simulink model "speed_control_disc_mpc"  (R2024a)
settings: Solver=VariableStepAuto  StartTime=0.0  StopTime=150  MaxStep=0.01  RelTol=1e-3
values from neighbouring files (symbols this model uses):
  F_max = 15    [init.m]
  F_min = -15    [init.m]
  K = ki*tau - kd/tau    (= -49.7)    [init.m]
  k = 0.5    [init.m]
  kbc = 1/(kp+kd/tau)    (= 0.0142857142857)    [init.m]
  kd = 5    [init.m]
  ki = 3    [init.m]
  kp = 20    [init.m]
  m = 10    [init.m]
  T = 0.1    [init.m]
  tau = 0.1    [init.m]
undefined symbols (not defined in the file or in its folder): DiscIntNeverNeededParam
libraries: simulink x4, mpclib x1, SignalEditorBlockLib x1
settings Model: Creator=berto  LastModifiedBy=berto

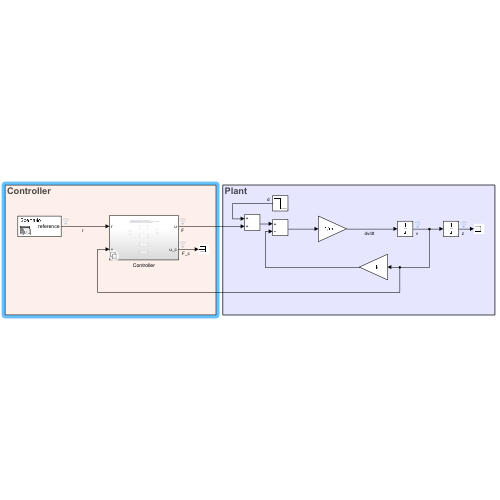
[thumbnail: Simulink's stored preview of the top-level diagram]
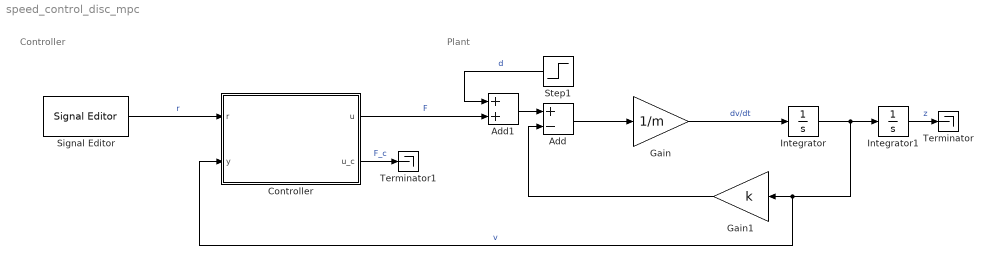
== system speed_control_disc_mpc ==
  note: Controller
  note: Plant
  Add : Sum  Inputs=+-
  Add1 : Sum
  Controller : Subsystem  Variant=on
  Gain : Gain  Gain=1/m
  Gain1 : Gain  Gain=k
  Integrator : Integrator
  Integrator1 : Integrator
  Signal Editor : SignalEditorBlockLib/Signal Editor  FileName=reference.mat  ActiveScenario=Scenario  ActiveSignal=reference  IsBus=off  OutputBusObjectStr=Bus: BusObject  SampleTime=0  ZeroCross=off  OutputAfterFinalValue=Setting to zero  Unit=inherit  PreserveSignalName=on  ApplySigPropsToAllScenarios=on  ApplySigPropsToAllSignals=off
  Step1 : Step  Time=120  After=-8  SampleTime=0
  Terminator : Terminator
  Terminator1 : Terminator
  wires:
  Controller/1(u) -> Add1/2  "F"
  Signal Editor/1 -> Controller/1(r)  "r"
  Add/1 -> Gain/1
  Gain/1 -> Integrator/1  "dv/dt"
  Integrator/1 -> Controller/2(y), Gain1/1, Integrator1/1  "v"
  Gain1/1 -> Add/2
  Step1/1 -> Add1/1  "d"
  Add1/1 -> Add/1
  Integrator1/1 -> Terminator/1  "z"
  Controller/2(u_c) -> Terminator1/1  "F_c"

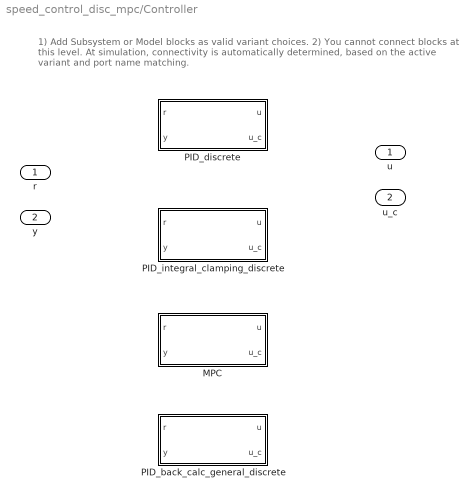
== system speed_control_disc_mpc/Controller ==
  note: 1) Add Subsystem or Model blocks as valid variant choices.
      | 2) You cannot connect blocks at this level. At simulation, connectivity is automatically
      | determined, based on the active variant and port name matching.
  r : Inport
  y : Inport  Port=2
  MPC : Subsystem  VariantControl=ctrl_type == 4
  PID_back_calc_general_discrete : Subsystem  VariantControl=ctrl_type == 3
  PID_discrete : Subsystem  VariantControl=ctrl_type == 0
  PID_integral_clamping_discrete : Subsystem  VariantControl=ctrl_type == 1
  u : Outport
  u_c : Outport  Port=2

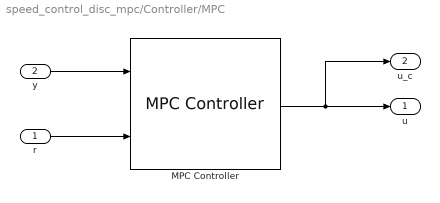
== system speed_control_disc_mpc/Controller/MPC ==
  r : Inport
  y : Inport  Port=2
  MPC Controller : mpclib/MPC Controller  SCDEnableBlockLinearizationSpecification=on  mpcobj=mpcobj  is_multiple=0  enable_value=0  return_u0=off  updateMPCinCallerWorkspace=on  md_inport=off  mv_inport=off  uref_inport=off  return_cost=off  return_mvseq=off  return_qpstatus=off  return_xseq=off  return_state=off  return_ovseq=off  state_inport=off  umin_inport=off  umax_inport=off  ymin_inport=off  ymax_inport=off  cc_inport=off  ywt_inport=off  uwt_inport=off  duwt_inport=off  rhoeps_inport=off  pm_inport=off  MaximumP=10  HorizonChoice=FixedHorizon  n_ts=1  n_p=10  n_mv=1  n_md=1  n_ud=0  n_mo=1  n_uo=0  BlockDataType=double  SampleTimeInherited=off  switch_inport=off
  u : Outport
  u_c : Outport  Port=2
  wires:
  MPC Controller/1 -> u_c/1, u/1
  r/1 -> MPC Controller/2
  y/1 -> MPC Controller/1

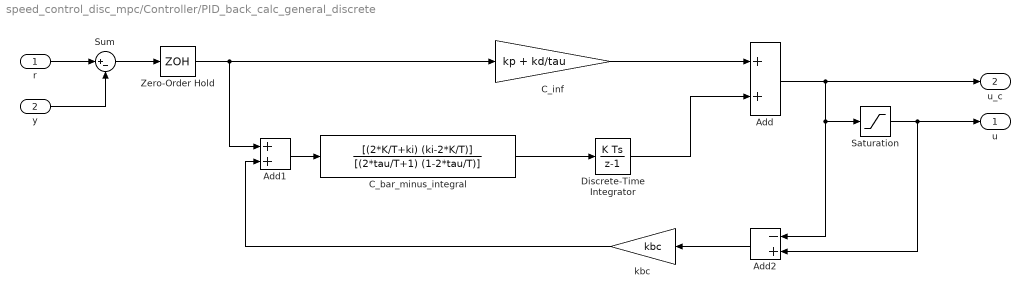
== system speed_control_disc_mpc/Controller/PID_back_calc_general_discrete ==
  r : Inport
  y : Inport  Port=2
  Add : Sum
  Add1 : Sum
  Add2 : Sum  Inputs=-+
  C_bar_minus_integral : DiscreteTransferFcn  Numerator=[(2*K/T+ki) (ki-2*K/T)]  Denominator=[(2*tau/T+1) (1-2*tau/T)]
  C_inf : Gain  Gain=kp + kd/tau
  Discrete-Time Integrator : DiscreteIntegrator  SampleTime=T  ICPrevOutput=DiscIntNeverNeededParam  ICPrevScaledInput=DiscIntNeverNeededParam
  Saturation : Saturate  UpperLimit=F_max  LowerLimit=F_min
  Sum : Sum  Inputs=|+-
  Zero-Order Hold : ZeroOrderHold  SampleTime=T
  kbc : Gain  Gain=kbc
  u : Outport
  u_c : Outport  Port=2
  wires:
  Add1/1 -> C_bar_minus_integral/1
  C_inf/1 -> Add/1
  kbc/1 -> Add1/2
  Add2/1 -> kbc/1
  Saturation/1 -> u/1, Add2/2
  Sum/1 -> Zero-Order Hold/1
  Add/1 -> Saturation/1, Add2/1, u_c/1
  Zero-Order Hold/1 -> C_inf/1, Add1/1
  C_bar_minus_integral/1 -> Discrete-Time Integrator/1
  Discrete-Time Integrator/1 -> Add/2
  r/1 -> Sum/1
  y/1 -> Sum/2

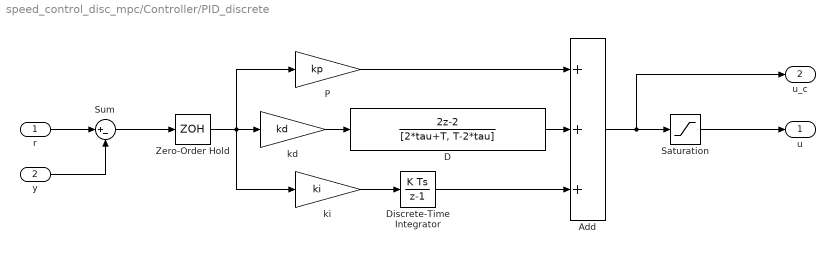
== system speed_control_disc_mpc/Controller/PID_discrete ==
  r : Inport
  y : Inport  Port=2
  Add : Sum  Inputs=+++
  D : DiscreteTransferFcn  Numerator=[2, -2]  Denominator=[2*tau+T, T-2*tau]
  Discrete-Time Integrator : DiscreteIntegrator  SampleTime=T  ICPrevOutput=DiscIntNeverNeededParam  ICPrevScaledInput=DiscIntNeverNeededParam
  P : Gain  Gain=kp
  Saturation : Saturate  UpperLimit=F_max  LowerLimit=F_min
  Sum : Sum  Inputs=|+-
  Zero-Order Hold : ZeroOrderHold  SampleTime=T
  kd : Gain  Gain=kd
  ki : Gain  Gain=ki
  u : Outport
  u_c : Outport  Port=2
  wires:
  ki/1 -> Discrete-Time Integrator/1
  Add/1 -> u_c/1, Saturation/1
  D/1 -> Add/2
  Discrete-Time Integrator/1 -> Add/3
  P/1 -> Add/1
  Sum/1 -> Zero-Order Hold/1
  Saturation/1 -> u/1
  Zero-Order Hold/1 -> kd/1, ki/1, P/1
  kd/1 -> D/1
  r/1 -> Sum/1
  y/1 -> Sum/2

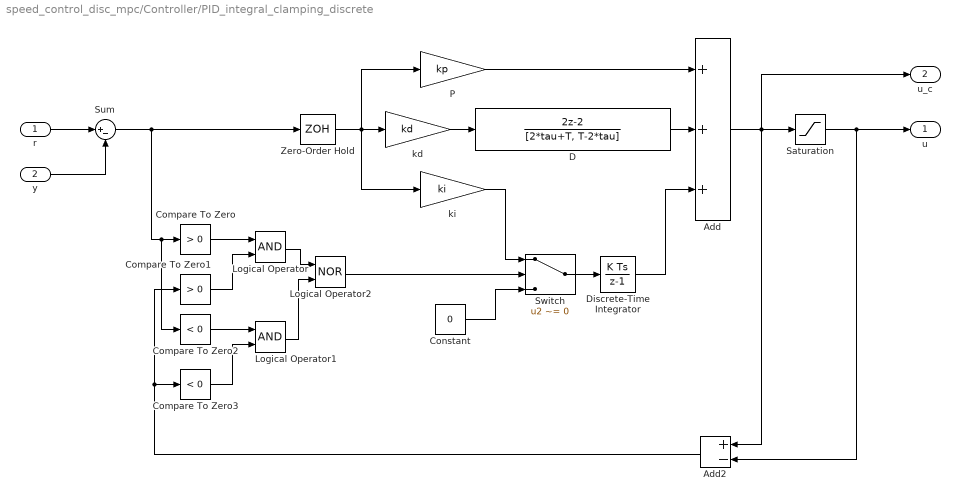
== system speed_control_disc_mpc/Controller/PID_integral_clamping_discrete ==
  r : Inport
  y : Inport  Port=2
  Add : Sum  Inputs=+++
  Add2 : Sum  Inputs=+-
  Compare To Zero : simulink/Logic and Bit Operations/Compare To Zero  relop=>  OutDataTypeStr=boolean
  Compare To Zero1 : simulink/Logic and Bit Operations/Compare To Zero  relop=>  OutDataTypeStr=boolean
  Compare To Zero2 : simulink/Logic and Bit Operations/Compare To Zero  relop=<  OutDataTypeStr=boolean
  Compare To Zero3 : simulink/Logic and Bit Operations/Compare To Zero  relop=<  OutDataTypeStr=boolean
  Constant : Constant  Value=0
  D : DiscreteTransferFcn  Numerator=[2, -2]  Denominator=[2*tau+T, T-2*tau]
  Discrete-Time Integrator : DiscreteIntegrator  SampleTime=T  ICPrevOutput=DiscIntNeverNeededParam  ICPrevScaledInput=DiscIntNeverNeededParam
  Logical Operator : Logic  AllPortsSameDT=off  OutDataTypeStr=boolean
  Logical Operator1 : Logic  AllPortsSameDT=off  OutDataTypeStr=boolean
  Logical Operator2 : Logic  Operator=NOR  AllPortsSameDT=off  OutDataTypeStr=boolean
  P : Gain  Gain=kp
  Saturation : Saturate  UpperLimit=F_max  LowerLimit=F_min
  Sum : Sum  Inputs=|+-
  Switch : Switch  Criteria=u2 ~= 0  SaturateOnIntegerOverflow=off  InputSameDT=off
  Zero-Order Hold : ZeroOrderHold  SampleTime=T
  kd : Gain  Gain=kd
  ki : Gain  Gain=ki
  u : Outport
  u_c : Outport  Port=2
  wires:
  Discrete-Time Integrator/1 -> Add/3
  Zero-Order Hold/1 -> kd/1, ki/1, P/1
  Sum/1 -> Compare To Zero2/1, Compare To Zero/1, Zero-Order Hold/1
  P/1 -> Add/1
  D/1 -> Add/2
  kd/1 -> D/1
  Switch/1 -> Discrete-Time Integrator/1
  ki/1 -> Switch/1
  Constant/1 -> Switch/3
  Saturation/1 -> Add2/2, u/1
  Add/1 -> Add2/1, u_c/1, Saturation/1
  Compare To Zero/1 -> Logical Operator/1
  Compare To Zero1/1 -> Logical Operator/2
  Add2/1 -> Compare To Zero3/1, Compare To Zero1/1
  Compare To Zero2/1 -> Logical Operator1/1
  Compare To Zero3/1 -> Logical Operator1/2
  Logical Operator/1 -> Logical Operator2/1
  Logical Operator1/1 -> Logical Operator2/2
  Logical Operator2/1 -> Switch/2
  r/1 -> Sum/1
  y/1 -> Sum/2
